simulink model "Assembly_union"  (R2020a)
(part 35 of 36)

  "IW{8,7}(9,:)'" : Constant  Value=[0.000434664733577357791961814914571959889144636690616607666015625;0.045556347475400903179743039572713314555585384368896484375;-0.08255063917253424587983090532361529767513275146484375;-0.1829786858408128102926326619126484729349613189697265625;-0.211050851458800148297001442188047803938388824462890625;0.2098187094850106071408646357667748816311359405517578125;0.241498469857383823988783433378557674586772918701171875;0.282869137888617228071552744950167834758758544921875;0.1613136878756551428892862531938590109348297119140625;-0.026180299976986086407659826136296032927930355072021484375;-0.309253299620219246346408681347384117543697357177734375;0.2464873134639166962767120594435255043208599090576171875;0.1439176436272844583630359238668461330235004425048828125;0.08492697485132182089184738060794188641011714935302734375;0.2224476745356778195628066896460950374603271484375;-0.08029734143684562341913846239549457095563411712646484375;0.1426464016313360450016745062384870834648609161376953125;-0.251210547864632649517346862921840511262416839599609375;0.2270650223014366309026712542618042789399623870849609375;-0.0636316274488852584578779669755022041499614715576171875;0.0723940392003423471845025005677598528563976287841796875;0.2108759012178855751784567473805509507656097412109375;-0.2659521337238299754091030990821309387683868408203125;0.210931337115611794441605297834030352532863616943359375;-0.2293028268875427766460006751003675162792205810546875;-0.25742263908987561560337553601129911839962005615234375;-0.21629239440297143293179260581382550299167633056640625;0.074883979272139189475865350686945021152496337890625;0.1832161367786570294047265861081541515886783599853515625;-0.138287143019176050895424623377039097249507904052734375;0.18430646189885913077688428529654629528522491455078125;-0.237663774024570895182506546916556544601917266845703125;-0.2266187718272578421885299349014530889689922332763671875;0.047815048590189014598994532434517168439924716949462890625;-0.263288898172046426093828586090239696204662322998046875;0.225784514533588775986316932176123373210430145263671875;-0.0258884125638330388208263599381098174490034580230712890625;-0.03848126503467096115596035588168888352811336517333984375;-0.046525940948262865803908283623968600295484066009521484375;-0.15446611258031339719565266932477243244647979736328125;-0.127937621017303937431819349512807093560695648193359375;0.256811630418195047109719553191098384559154510498046875;0.07276296691673396488386771352452342398464679718017578125;-0.06527848078427030131809516433349926955997943878173828125;-0.01368189203072979302777678611846567946486175060272216796875;0.02070468861066199206533156029763631522655487060546875;0.30359986596022714433473765893722884356975555419921875;0.002494768556101998289997734303824472590349614620208740234375;0.1448279081807268553472312078156392090022563934326171875;-0.22959288214594664179202254672418348491191864013671875;0.282806364126715059637007243509287945926189422607421875;0.060910430085892038054584674000579980202019214630126953125;0.0816954496177734468265185796553851105272769927978515625;-0.00551188698131989569806155060405217227526009082794189453125;-0.11882811018164039784661412113564438186585903167724609375;-0.044807485028413862604423911761841736733913421630859375;-0.213491342725472710295520073486841283738613128662109375;0.2314953621249038751006565917123225517570972442626953125;0.214180107827206589465873776134685613214969635009765625;-0.264366588888496234499569936815532855689525604248046875;-0.19055260714008259714802306916681118309497833251953125;0.1850524193117057125679281170960166491568088531494140625;-0.08132623138830406828159169663194916211068630218505859375;-0.291562579915350561510223315053735859692096710205078125;0.08645125927600004478446038547190255485475063323974609375;-0.245638445307413577634036982999532483518123626708984375;-0.1805853084085567161753971276993979699909687042236328125;-0.057074161075482431060290622326647280715405941009521484375;0.166263596844649363948320797135238535702228546142578125;-0.22020611068891593475882473285309970378875732421875]
      mask Display: e = 0.06;c1 = [120 150 230]/255;c2 = ([120 150 230]+0)/383;c3 = ([120 150 230]+128)/383;patch([0 1 1 0],[0 0 1 1],c1);patch([0 1 1 1-e 1-e 0+e],[0 0 1 1-e 0+e 0+e],c2);patch([0 0 1 1-e 0+e 0+e],[0 1 1 1-e 1-e 0+e],c3);plot([0 1 1 0 0],[0 0 1 1 0]);disp('weights');
  Mux : Mux  Inputs=63
      mask Display: e = 0.06;c1 = [120 150 230]/255;c2 = ([120 150 230]+0)/383;c3 = ([120 150 230]+128)/383;patch([0 1 1 0],[0 0 1 1],c1);patch([0 1 1 1-e 1-e 0+e],[0 0 1 1-e 0+e 0+e],c2);patch([0 0 1 1-e 0+e 0+e],[0 1 1 1-e 1-e 0+e],c3);plot([0 1 1 0 0],[0 0 1 1 0]);disp('Mux');
  dotprod{1..63} (63 alike) : neural/Weight Functions/dotprod
  "lz{8,7}" : Outport
      mask Display: e = 0.06;c1 = [120 230 180]/255;c2 = ([120 230 180]+0)/(256+128);c3 = ([120 230 180]+128)/(256+128);patch([0 1 1 0],[0 0 1 1],c1);patch([0 1 1 1-e 1-e 0+e],[0 0 1 1-e 0+e 0+e],c2);patch([0 0 1 1-e 0+e 0+e],[0 1 1 1-e 1-e 0+e],c3);plot([0 1 1 0 0],[0 0 1 1 0]);
  wires:
  "IW{8,7}(1,:)'"/1 -> dotprod1/1
  "ad{8,7}"/1 -> dotprod1/2, dotprod2/2, dotprod3/2, dotprod4/2, dotprod5/2, dotprod6/2, dotprod7/2, dotprod8/2, dotprod9/2, dotprod10/2, dotprod11/2, dotprod12/2, dotprod13/2, dotprod14/2, dotprod15/2, dotprod16/2, dotprod17/2, dotprod18/2, dotprod19/2, dotprod20/2, dotprod21/2, dotprod22/2, dotprod23/2, dotprod24/2, dotprod25/2, dotprod26/2, dotprod27/2, dotprod28/2, dotprod29/2, dotprod30/2, dotprod31/2, dotprod32/2, dotprod33/2, dotprod34/2, dotprod35/2, dotprod36/2, dotprod37/2, dotprod38/2, dotprod39/2, dotprod40/2, dotprod41/2, dotprod42/2, dotprod43/2, dotprod44/2, dotprod45/2, dotprod46/2, dotprod47/2, dotprod48/2, dotprod49/2, dotprod50/2, dotprod51/2, dotprod52/2, dotprod53/2, dotprod54/2, dotprod55/2, dotprod56/2, dotprod57/2, dotprod58/2, dotprod59/2, dotprod60/2, dotprod61/2, dotprod62/2, dotprod63/2
  dotprod1/1 -> Mux/1
  "IW{8,7}(2,:)'"/1 -> dotprod2/1
  dotprod2/1 -> Mux/2
  "IW{8,7}(3,:)'"/1 -> dotprod3/1
  dotprod3/1 -> Mux/3
  "IW{8,7}(4,:)'"/1 -> dotprod4/1
  dotprod4/1 -> Mux/4
  "IW{8,7}(5,:)'"/1 -> dotprod5/1
  dotprod5/1 -> Mux/5
  "IW{8,7}(6,:)'"/1 -> dotprod6/1
  dotprod6/1 -> Mux/6
  "IW{8,7}(7,:)'"/1 -> dotprod7/1
  dotprod7/1 -> Mux/7
  "IW{8,7}(8,:)'"/1 -> dotprod8/1
  dotprod8/1 -> Mux/8
  "IW{8,7}(9,:)'"/1 -> dotprod9/1
  dotprod9/1 -> Mux/9
  "IW{8,7}(10,:)'"/1 -> dotprod10/1
  dotprod10/1 -> Mux/10
  "IW{8,7}(11,:)'"/1 -> dotprod11/1
  dotprod11/1 -> Mux/11
  "IW{8,7}(12,:)'"/1 -> dotprod12/1
  dotprod12/1 -> Mux/12
  "IW{8,7}(13,:)'"/1 -> dotprod13/1
  dotprod13/1 -> Mux/13
  "IW{8,7}(14,:)'"/1 -> dotprod14/1
  dotprod14/1 -> Mux/14
  "IW{8,7}(15,:)'"/1 -> dotprod15/1
  dotprod15/1 -> Mux/15
  "IW{8,7}(16,:)'"/1 -> dotprod16/1
  dotprod16/1 -> Mux/16
  "IW{8,7}(17,:)'"/1 -> dotprod17/1
  dotprod17/1 -> Mux/17
  "IW{8,7}(18,:)'"/1 -> dotprod18/1
  dotprod18/1 -> Mux/18
  "IW{8,7}(19,:)'"/1 -> dotprod19/1
  dotprod19/1 -> Mux/19
  "IW{8,7}(20,:)'"/1 -> dotprod20/1
  dotprod20/1 -> Mux/20
  "IW{8,7}(21,:)'"/1 -> dotprod21/1
  dotprod21/1 -> Mux/21
  "IW{8,7}(22,:)'"/1 -> dotprod22/1
  dotprod22/1 -> Mux/22
  "IW{8,7}(23,:)'"/1 -> dotprod23/1
  dotprod23/1 -> Mux/23
  "IW{8,7}(24,:)'"/1 -> dotprod24/1
  dotprod24/1 -> Mux/24
  "IW{8,7}(25,:)'"/1 -> dotprod25/1
  dotprod25/1 -> Mux/25
  "IW{8,7}(26,:)'"/1 -> dotprod26/1
  dotprod26/1 -> Mux/26
  "IW{8,7}(27,:)'"/1 -> dotprod27/1
  dotprod27/1 -> Mux/27
  "IW{8,7}(28,:)'"/1 -> dotprod28/1
  dotprod28/1 -> Mux/28
  "IW{8,7}(29,:)'"/1 -> dotprod29/1
  dotprod29/1 -> Mux/29
  "IW{8,7}(30,:)'"/1 -> dotprod30/1
  dotprod30/1 -> Mux/30
  "IW{8,7}(31,:)'"/1 -> dotprod31/1
  dotprod31/1 -> Mux/31
  "IW{8,7}(32,:)'"/1 -> dotprod32/1
  dotprod32/1 -> Mux/32
  "IW{8,7}(33,:)'"/1 -> dotprod33/1
  dotprod33/1 -> Mux/33
  "IW{8,7}(34,:)'"/1 -> dotprod34/1
  dotprod34/1 -> Mux/34
  "IW{8,7}(35,:)'"/1 -> dotprod35/1
  dotprod35/1 -> Mux/35
  "IW{8,7}(36,:)'"/1 -> dotprod36/1
  dotprod36/1 -> Mux/36
  "IW{8,7}(37,:)'"/1 -> dotprod37/1
  dotprod37/1 -> Mux/37
  "IW{8,7}(38,:)'"/1 -> dotprod38/1
  dotprod38/1 -> Mux/38
  "IW{8,7}(39,:)'"/1 -> dotprod39/1
  dotprod39/1 -> Mux/39
  "IW{8,7}(40,:)'"/1 -> dotprod40/1
  dotprod40/1 -> Mux/40
  "IW{8,7}(41,:)'"/1 -> dotprod41/1
  dotprod41/1 -> Mux/41
  "IW{8,7}(42,:)'"/1 -> dotprod42/1
  dotprod42/1 -> Mux/42
  "IW{8,7}(43,:)'"/1 -> dotprod43/1
  dotprod43/1 -> Mux/43
  "IW{8,7}(44,:)'"/1 -> dotprod44/1
  dotprod44/1 -> Mux/44
  "IW{8,7}(45,:)'"/1 -> dotprod45/1
  dotprod45/1 -> Mux/45
  "IW{8,7}(46,:)'"/1 -> dotprod46/1
  dotprod46/1 -> Mux/46
  "IW{8,7}(47,:)'"/1 -> dotprod47/1
  dotprod47/1 -> Mux/47
  "IW{8,7}(48,:)'"/1 -> dotprod48/1
  dotprod48/1 -> Mux/48
  "IW{8,7}(49,:)'"/1 -> dotprod49/1
  dotprod49/1 -> Mux/49
  "IW{8,7}(50,:)'"/1 -> dotprod50/1
  dotprod50/1 -> Mux/50
  "IW{8,7}(51,:)'"/1 -> dotprod51/1
  dotprod51/1 -> Mux/51
  "IW{8,7}(52,:)'"/1 -> dotprod52/1
  dotprod52/1 -> Mux/52
  "IW{8,7}(53,:)'"/1 -> dotprod53/1
  dotprod53/1 -> Mux/53
  "IW{8,7}(54,:)'"/1 -> dotprod54/1
  dotprod54/1 -> Mux/54
  "IW{8,7}(55,:)'"/1 -> dotprod55/1
  dotprod55/1 -> Mux/55
  "IW{8,7}(56,:)'"/1 -> dotprod56/1
  dotprod56/1 -> Mux/56
  "IW{8,7}(57,:)'"/1 -> dotprod57/1
  dotprod57/1 -> Mux/57
  "IW{8,7}(58,:)'"/1 -> dotprod58/1
  dotprod58/1 -> Mux/58
  "IW{8,7}(59,:)'"/1 -> dotprod59/1
  dotprod59/1 -> Mux/59
  "IW{8,7}(60,:)'"/1 -> dotprod60/1
  dotprod60/1 -> Mux/60
  "IW{8,7}(61,:)'"/1 -> dotprod61/1
  dotprod61/1 -> Mux/61
  "IW{8,7}(62,:)'"/1 -> dotprod62/1
  dotprod62/1 -> Mux/62
  "IW{8,7}(63,:)'"/1 -> dotprod63/1
  dotprod63/1 -> Mux/63
  Mux/1 -> "lz{8,7}"/1
